simulink model "exp2_task2_three_point_model"  (R2024a)
settings: Solver=ode45  StartTime=0.0  StopTime=10  MaxStep=0.01  RelTol=1e-3
InitFcn:
  | exp3_task('init','三点法')
values from neighbouring files (symbols this model uses):
  par = [P.v; P.vT; P.r0; P.q0; P.xT0; P.yT0; P.HIT; P.K;         P.sigmaT; P.sigmaM0; P.g0; P.tmax]    [exp3_task.m]    (also in export_workspace_to_csv.m = evalin('base', 'par'))
  x0 = [0; 0; P.sigmaM0; 0]    [exp3_task.m]
settings Model: Creator=taole  LastModifiedBy=taole

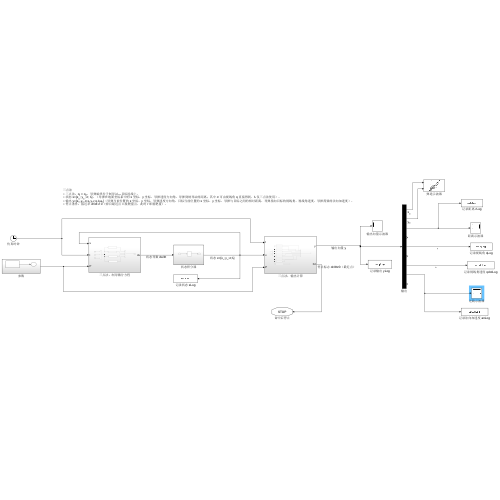
[thumbnail: Simulink's stored preview of the top-level diagram]
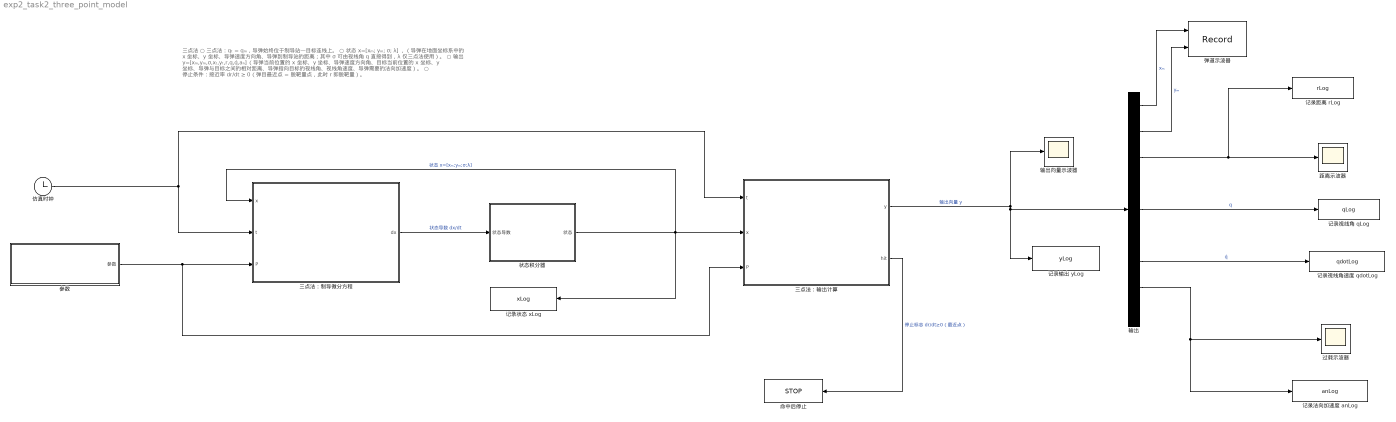
== system exp2_task2_three_point_model ==
  note: 三点法
      | ○ 三点法：qₜ = qₘ，导弹始终位于制导站—目标连线上。
      | ○ 状态 x=[xₘ; yₘ; σ; λ]，（导弹在地面坐标系中的 x 坐标、y 坐标、导弹速度方向角、导弹到制导站的距离；其中 σ 可由视线角 q 直接得到，λ 仅三点法使用）。
      | ○ 输出 y=[xₘ,yₘ,σ,xₜ,yₜ,r,q,q̇,aₙ]（导弹当前位置的 x 坐标、y 坐标、导弹速度方向角、目标当前位置的 x 坐标、y 坐标、导弹与目标之间的相对距离、导弹指向目标的视线角、视线角速度、导弹需要的法向加速度）。
      | ○ 停止条件：接近率 dr/dt ≥ 0（弹目最近点 = 脱靶量点，此时 r 即脱靶量）。
  三点法：制导微分方程 : Subsystem
  三点法：输出计算 : Subsystem
  仿真时钟 : Clock
  参数 : Subsystem
  命中后停止 : Stop
  弹道示波器 : Record  FileSettingsInternal="{\"entries\":[{\"content\":{\"excelSettings\":{\"content\":{},\"type\":\"Streamout.ExcelSettings\"}},\"type\":\"Streamout.FileSettingStorage\",\"uuid\":\"\"}],\"packageUris\":[\"http:\\/\\/schema.mathworks.com\\/mf0\\/streamout_blocks\\/R2020a\"],\"version\":\"1.0\"}"  Layout=[1 1]  SignalsInternal="{\"entries\":[{\"content\":{\"signals\":[{\"content\":{\"blockPath\":[],\"dimensions\":[1],\"domain\":\"\",\"lineColor\":\"#7e2f8e\",\"lineWidth\":2,\"plots\":[ 1 ],\"port\":1,\"sid\":[\"\"],\"signalID\":1,\"signalName\":\"xₘ\"},\"type\":\"RecordBlkView.Signal\",\"uuid\":\"\"},{\"content\":{\"blockPath\":[],\"dimensions\":[1],\"domain\":\"\",\"lineColor\":\"#139fff\",\"plots\":[ 1 ],\"port\":2,\"sid\":[\"\"],\"signalID\":2,\"signalName\":\"yₘ\"},\"type\":\"RecordBlkView.Signal\",\"uuid\":\"\"}]},\"type\":\"RecordBlkView.InputSignals\",\"uuid\":\"\"}],\"packageUris\":[\"http:\\/\\/schema.mathworks.com\\/mf0\\/streamout_blocks\\/R2020a\"],\"version\":\"1.0\"}"  VisualizationBindings="{\"xyplotplugin\":{\"info\":[{\"series\":[{\"bindingParametersList\":[{\"parameter\":\"X-Axis\",\"signalID\":1,\"signalName\":\"xₘ\"},{\"parameter\":\"Y-Axis\",\"signalID\":2,\"signalName\":\"yₘ\"}],\"seriesID\":0}],\"subplotID\":1}]}}"  CompatibilityTag=XY
  状态积分器 : Subsystem
  记录法向加速度 anLog : ToWorkspace  VariableName=anLog  SaveFormat=Timeseries  SampleTime=-1
  记录状态 xLog : ToWorkspace  VariableName=xLog  SaveFormat=Timeseries  SampleTime=-1
  记录视线角 qLog : ToWorkspace  VariableName=qLog  SaveFormat=Timeseries  SampleTime=-1
  记录视线角速度 qdotLog : ToWorkspace  VariableName=qdotLog  SaveFormat=Timeseries  SampleTime=-1
  记录距离 rLog : ToWorkspace  VariableName=rLog  SaveFormat=Timeseries  SampleTime=-1
  记录输出 yLog : ToWorkspace  VariableName=yLog  SaveFormat=Timeseries  SampleTime=-1
  距离示波器 : Scope
  输出 : Demux  Outputs=9
  输出向量示波器 : Scope
  过载示波器 : Scope
  wires:
  仿真时钟/1 -> 三点法：输出计算/1(t), 三点法：制导微分方程/2(t)
  参数/1(参数) -> 三点法：输出计算/3(P), 三点法：制导微分方程/3(P)
  三点法：制导微分方程/1(dx) -> 状态积分器/1(状态导数)  "状态导数 dx/dt"
  状态积分器/1(状态) -> 三点法：制导微分方程/1(x), 三点法：输出计算/2(x), 记录状态 xLog/1  "状态 x=[xₘ;yₘ;σ;λ]"
  三点法：输出计算/1(y) -> 记录输出 yLog/1, 输出/1, 输出向量示波器/1  "输出向量 y"
  输出/1 -> 弹道示波器/1  "xₘ"
  输出/2 -> 弹道示波器/2  "yₘ"
  三点法：输出计算/2(hit) -> 命中后停止/1  "停止标志 dr/dt≥0（最近点）"
  输出/3 -> 记录距离 rLog/1, 距离示波器/1
  输出/5 -> 记录视线角 qLog/1  "q"
  输出/7 -> 记录视线角速度 qdotLog/1  "q̇"
  输出/8 -> 记录法向加速度 anLog/1, 过载示波器/1

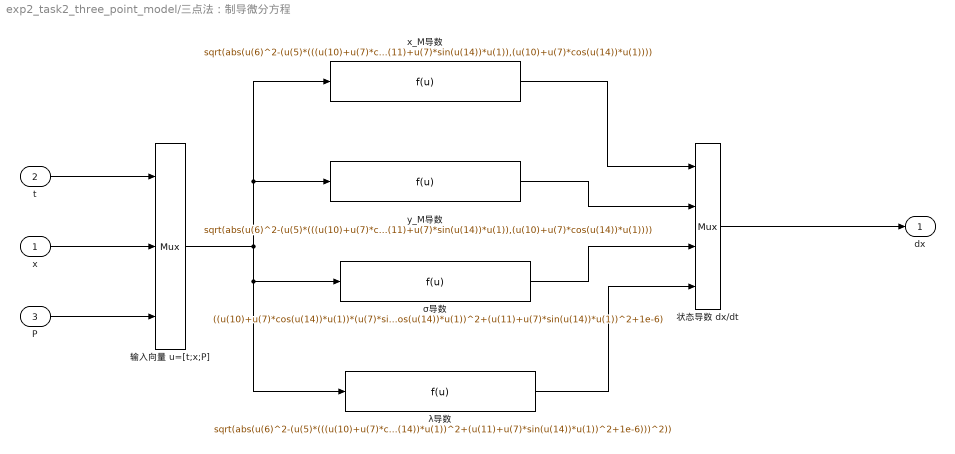
== system exp2_task2_three_point_model/三点法：制导微分方程 ==
  x : Inport
  t : Inport  Port=2
  P : Inport  Port=3
  x_M导数 : Fcn  Expr=sqrt(abs(u(6)^2-(u(5)*(((u(10)+u(7)*cos(u(14))*u(1))*(u(7)*sin(u(14)))-(u(11)+u(7)*sin(u(14))*u(1))*(u(7)*cos(u(14))))/((u(10)+u(7)*cos(u(14))*u(1))^2+(u(11)+u(7)*sin(u(14))*u(1))^2+1e-6)))^2))*cos(atan2((u(11)+u(7)*sin(u(14))*u(1)),(u(10)+u(7)*cos(u(14))*u(1))))-u(5)*(((u(10)+u(7)*cos(u(14))*u(1))*(u(7)*sin(u(14)))-(u(11)+u(7)*sin(u(14))*u(1))*(u(7)*cos(u(14))))/((u(10)+u(7)*cos(u(14))*u(1))^2+(u(11)+u(7)*sin(u(14))*u(1))^2+1e-6))*sin(atan2((u(11)+u(7)*sin(u(14))*u(1)),(u(10)+u(7)*cos(u(14))*u(1))))
  y_M导数 : Fcn  Expr=sqrt(abs(u(6)^2-(u(5)*(((u(10)+u(7)*cos(u(14))*u(1))*(u(7)*sin(u(14)))-(u(11)+u(7)*sin(u(14))*u(1))*(u(7)*cos(u(14))))/((u(10)+u(7)*cos(u(14))*u(1))^2+(u(11)+u(7)*sin(u(14))*u(1))^2+1e-6)))^2))*sin(atan2((u(11)+u(7)*sin(u(14))*u(1)),(u(10)+u(7)*cos(u(14))*u(1))))+u(5)*(((u(10)+u(7)*cos(u(14))*u(1))*(u(7)*sin(u(14)))-(u(11)+u(7)*sin(u(14))*u(1))*(u(7)*cos(u(14))))/((u(10)+u(7)*cos(u(14))*u(1))^2+(u(11)+u(7)*sin(u(14))*u(1))^2+1e-6))*cos(atan2((u(11)+u(7)*sin(u(14))*u(1)),(u(10)+u(7)*cos(u(14))*u(1))))
  λ导数 : Fcn  Expr=sqrt(abs(u(6)^2-(u(5)*(((u(10)+u(7)*cos(u(14))*u(1))*(u(7)*sin(u(14)))-(u(11)+u(7)*sin(u(14))*u(1))*(u(7)*cos(u(14))))/((u(10)+u(7)*cos(u(14))*u(1))^2+(u(11)+u(7)*sin(u(14))*u(1))^2+1e-6)))^2))
  σ导数 : Fcn  Expr=((u(10)+u(7)*cos(u(14))*u(1))*(u(7)*sin(u(14)))-(u(11)+u(7)*sin(u(14))*u(1))*(u(7)*cos(u(14))))/((u(10)+u(7)*cos(u(14))*u(1))^2+(u(11)+u(7)*sin(u(14))*u(1))^2+1e-6)
  状态导数 dx/dt : Mux
  输入向量 u=[t;x;P] : Mux  Inputs=3
  dx : Outport
  wires:
  t/1 -> 输入向量 u=[t;x;P]/1
  x/1 -> 输入向量 u=[t;x;P]/2
  P/1 -> 输入向量 u=[t;x;P]/3
  输入向量 u=[t;x;P]/1 -> y_M导数/1, x_M导数/1, λ导数/1, σ导数/1
  x_M导数/1 -> 状态导数 dx/dt/1
  y_M导数/1 -> 状态导数 dx/dt/2
  σ导数/1 -> 状态导数 dx/dt/3
  λ导数/1 -> 状态导数 dx/dt/4
  状态导数 dx/dt/1 -> dx/1

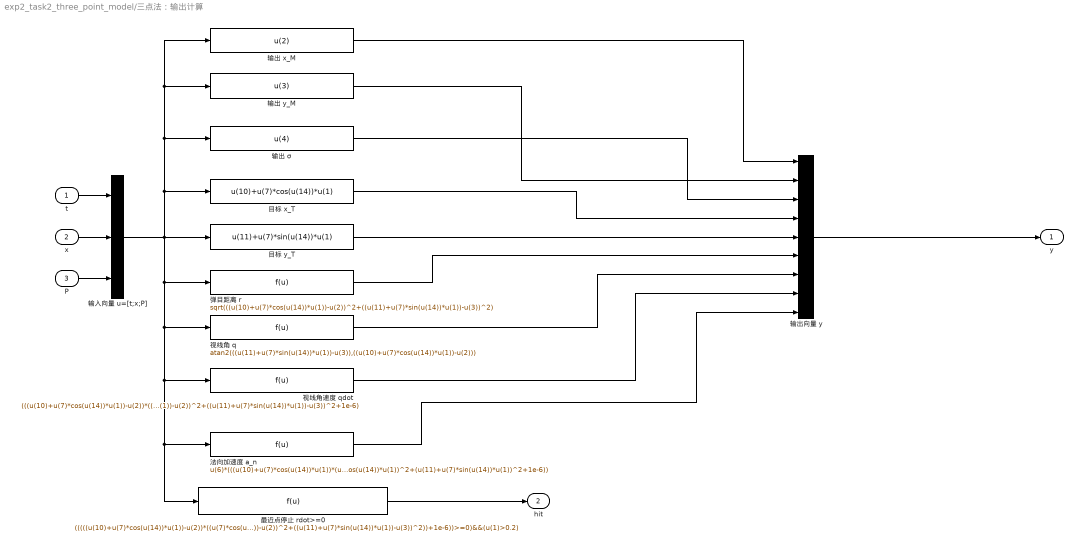
== system exp2_task2_three_point_model/三点法：输出计算 ==
  t : Inport
  x : Inport  Port=2
  P : Inport  Port=3
  弹目距离 r : Fcn  Expr=sqrt(((u(10)+u(7)*cos(u(14))*u(1))-u(2))^2+((u(11)+u(7)*sin(u(14))*u(1))-u(3))^2)
  最近点停止 rdot>=0 : Fcn  Expr=(((((u(10)+u(7)*cos(u(14))*u(1))-u(2))*((u(7)*cos(u(14)))-((sqrt(abs(u(6)^2-(u(5)*(((u(10)+u(7)*cos(u(14))*u(1))*(u(7)*sin(u(14)))-(u(11)+u(7)*sin(u(14))*u(1))*(u(7)*cos(u(14))))/((u(10)+u(7)*cos(u(14))*u(1))^2+(u(11)+u(7)*sin(u(14))*u(1))^2+1e-6)))^2)))*cos(atan2((u(11)+u(7)*sin(u(14))*u(1)),(u(10)+u(7)*cos(u(14))*u(1))))-u(5)*(((u(10)+u(7)*cos(u(14))*u(1))*(u(7)*sin(u(14)))-(u(11)+u(7)*sin(u(14))*u(1))*(u(7)*cos(u(14))))/((u(10)+u(7)*cos(u(14))*u(1))^2+(u(11)+u(7)*sin(u(14))*u(1))^2+1e-6))*sin(atan2((u(11)+u(7)*sin(u(14))*u(1)),(u(10)+u(7)*cos(u(14))*u(1))))))+((u(11)+u(7)*sin(u(14))*u(1))-u(3))*((u(7)*sin(u(14)))-((sqrt(abs(u(6)^2-(u(5)*(((u(10)+u(7)*cos(u(14))*u(1))*(u(7)*sin(u(14)))-(u(11)+u(7)*sin(u(14))*u(1))*(u(7)*cos(u(14))))/((u(10)+u(7)*cos(u(14))*u(1))^2+(u(11)+u(7)*sin(u(14))*u(1))^2+1e-6)))^2)))*sin(atan2((u(11)+u(7)*sin(u(14))*u(1)),(u(10)+u(7)*cos(u(14))*u(1))))+u(5)*(((u(10)+u(7)*cos(u(14))*u(1))*(u(7)*sin(u(14)))-(u(11)+u(7)*sin(u(14))*u(1))*(u(7)*cos(u(14))))/((u(10)+u(7)*cos(u(14))*u(1))^2+(u(11)+u(7)*sin(u(14))*u(1))^2+1e-6))*cos(atan2((u(11)+u(7)*sin(u(14))*u(1)),(u(10)+u(7)*cos(u(14))*u(1)))))))/((sqrt(((u(10)+u(7)*cos(u(14))*u(1))-u(2))^2+((u(11)+u(7)*sin(u(14))*u(1))-u(3))^2))+1e-6))>=0)&&(u(1)>0.2)
  法向加速度 a_n : Fcn  Expr=u(6)*(((u(10)+u(7)*cos(u(14))*u(1))*(u(7)*sin(u(14)))-(u(11)+u(7)*sin(u(14))*u(1))*(u(7)*cos(u(14))))/((u(10)+u(7)*cos(u(14))*u(1))^2+(u(11)+u(7)*sin(u(14))*u(1))^2+1e-6))
  目标 x_T : Fcn  Expr=u(10)+u(7)*cos(u(14))*u(1)
  目标 y_T : Fcn  Expr=u(11)+u(7)*sin(u(14))*u(1)
  视线角 q : Fcn  Expr=atan2(((u(11)+u(7)*sin(u(14))*u(1))-u(3)),((u(10)+u(7)*cos(u(14))*u(1))-u(2)))
  视线角速度 qdot : Fcn  Expr=(((u(10)+u(7)*cos(u(14))*u(1))-u(2))*((u(7)*sin(u(14)))-(u(6)*sin(u(4))))-((u(11)+u(7)*sin(u(14))*u(1))-u(3))*((u(7)*cos(u(14)))-(u(6)*cos(u(4)))))/(((u(10)+u(7)*cos(u(14))*u(1))-u(2))^2+((u(11)+u(7)*sin(u(14))*u(1))-u(3))^2+1e-6)
  输入向量 u=[t;x;P] : Mux  Inputs=3
  输出 x_M : Fcn  Expr=u(2)
  输出 y_M : Fcn  Expr=u(3)
  输出 σ : Fcn  Expr=u(4)
  输出向量 y : Mux  Inputs=9
  y : Outport
  hit : Outport  Port=2
  wires:
  t/1 -> 输入向量 u=[t;x;P]/1
  x/1 -> 输入向量 u=[t;x;P]/2
  P/1 -> 输入向量 u=[t;x;P]/3
  输入向量 u=[t;x;P]/1 -> 法向加速度 a_n/1, 最近点停止 rdot>=0/1, 视线角速度 qdot/1, 视线角 q/1, 弹目距离 r/1, 目标 y_T/1, 输出 σ/1, 输出 x_M/1, 输出 y_M/1, 目标 x_T/1
  输出 x_M/1 -> 输出向量 y/1
  输出 y_M/1 -> 输出向量 y/2
  输出 σ/1 -> 输出向量 y/3
  目标 x_T/1 -> 输出向量 y/4
  目标 y_T/1 -> 输出向量 y/5
  弹目距离 r/1 -> 输出向量 y/6
  视线角 q/1 -> 输出向量 y/7
  视线角速度 qdot/1 -> 输出向量 y/8
  法向加速度 a_n/1 -> 输出向量 y/9
  输出向量 y/1 -> y/1
  最近点停止 rdot>=0/1 -> hit/1

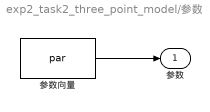
== system exp2_task2_three_point_model/参数 ==
  参数向量 : Constant  Value=par
  参数 : Outport
  wires:
  参数向量/1 -> 参数/1

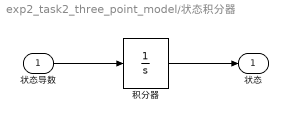
== system exp2_task2_three_point_model/状态积分器 ==
  状态导数 : Inport
  积分器 : Integrator  InitialCondition=x0
  状态 : Outport
  wires:
  状态导数/1 -> 积分器/1
  积分器/1 -> 状态/1
